simulink model "P1_son"  (R2021b)
settings: Solver=VariableStepAuto  StartTime=0.0  StopTime=10.0  RelTol=1e-3
values from neighbouring files (symbols this model uses):
  C = [cs -cs;-cs cs]    [P1_Fre_Response_m.m]
  invM = inv(M)    [P1_Fre_Response_m.m]
  K = [ks -ks;-ks ks+ku]    [P1_Fre_Response_m.m]
  Y = [0;ku]    [P1_Fre_Response_m.m]
settings Model: Creator=11639  LastModifiedBy=11639

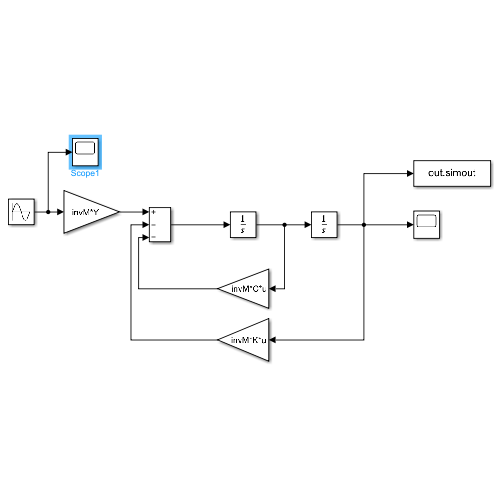
[thumbnail: Simulink's stored preview of the top-level diagram]
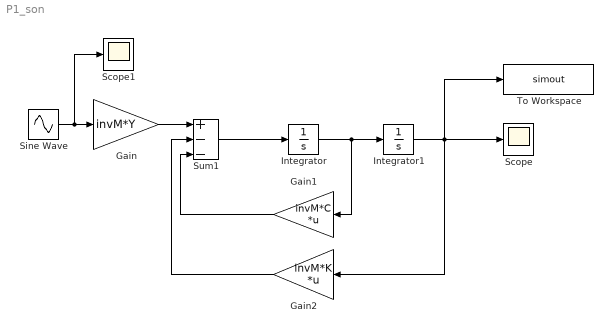
== system P1_son ==
  Gain : Gain  Gain=invM*Y
  Gain1 : Gain  Gain=invM*C  Multiplication=Matrix(K*u)
  Gain2 : Gain  Gain=invM*K  Multiplication=Matrix(K*u)
  Integrator : Integrator
  Integrator1 : Integrator
  Scope : Scope
  Scope1 : Scope
  Sine Wave : Sin  SampleTime=0
  Sum1 : Sum  Inputs=+--
  To Workspace : ToWorkspace  VariableName=simout  SaveFormat=Timeseries  SampleTime=-1
  wires:
  Integrator/1 -> Gain1/1, Integrator1/1
  Sine Wave/1 -> Scope1/1, Gain/1
  Integrator1/1 -> To Workspace/1, Scope/1, Gain2/1
  Gain1/1 -> Sum1/3
  Gain/1 -> Sum1/1
  Sum1/1 -> Integrator/1
  Gain2/1 -> Sum1/2
